simulink model "phi_mu"  (R2022a)
settings: Solver=VariableStepAuto  StartTime=0.0  StopTime=30  RelTol=1e-3
undefined symbols (not defined in the file or in its folder): G_phi_samples
libraries: simulink x4, cstblocks x2
settings Model: Creator=persian  LastModifiedBy=persian

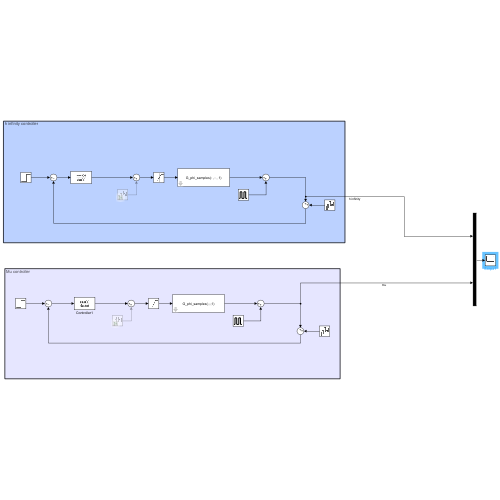
[thumbnail: Simulink's stored preview of the top-level diagram]
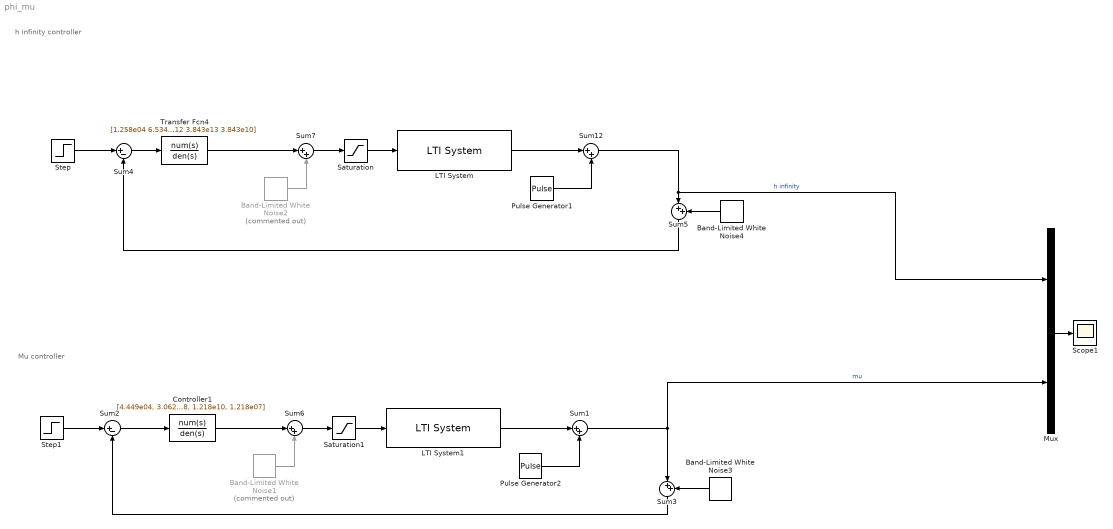
== system phi_mu ==
  note: h infinity controller
  note: Mu controller
  Band-Limited White Noise1 : simulink/Sources/Band-Limited White Noise  Commented=on  Cov=[0.001]  Ts=0.01  seed=[23341]
  Band-Limited White Noise2 : simulink/Sources/Band-Limited White Noise  Commented=on  Cov=[0.001]  Ts=0.01  seed=[23341]
  Band-Limited White Noise3 : simulink/Sources/Band-Limited White Noise  Cov=[0.0001]  Ts=0.01  seed=[23341]
  Band-Limited White Noise4 : simulink/Sources/Band-Limited White Noise  Cov=[0.0001]  Ts=0.01  seed=[23341]
  Controller1 : TransferFcn  Numerator=[4.449e04, 3.062e07, 8.69e08, 2.019e10, 1.453e11]  Denominator=[1, 3716, 2.98e06, 2.73e08, 1.218e10, 1.218e07]
  LTI System : cstblocks/LTI System  sys=G_phi_samples(: , : , 1)  IC=[]
  LTI System1 : cstblocks/LTI System  sys=G_phi_samples(:,:,1)  IC=[]
  Mux : Mux  Inputs=2
  Pulse Generator1 : DiscretePulseGenerator  PulseType=Time based  Amplitude=0.1  Period=1.5  PulseWidth=5
  Pulse Generator2 : DiscretePulseGenerator  PulseType=Time based  Amplitude=0.1  Period=1.5  PulseWidth=5
  Saturation : Saturate  UpperLimit=20  LowerLimit=-20
  Saturation1 : Saturate  UpperLimit=20  LowerLimit=-20
  Scope1 : Scope
  Step : Step  SampleTime=0
  Step1 : Step  SampleTime=0
  Sum{1,3,5..7,12} (6 alike) : Sum  Inputs=|++
  Sum2 : Sum  Inputs=|+-
  Sum4 : Sum  Inputs=|+-
  Transfer Fcn4 : TransferFcn  Numerator=[1.258e04 6.534e06 6.665e08 3.016e10 7.851e11 1.256e13 1.142e14 3.868e14]  Denominator=[1 2032 1.172e06 1.496e08 9.86e09 3.484e11 5.991e12 3.843e13 3.843e10]
  wires:
  Band-Limited White Noise1/1 -> Sum6/2
  Transfer Fcn4/1 -> Sum7/1
  Controller1/1 -> Sum6/1
  Band-Limited White Noise4/1 -> Sum5/2
  LTI System/1 -> Sum12/1
  Sum1/1 -> Mux/2, Sum3/1  "mu"
  Step/1 -> Sum4/1
  Band-Limited White Noise2/1 -> Sum7/2
  Sum7/1 -> Saturation/1
  Sum5/1 -> Sum4/2
  Sum4/1 -> Transfer Fcn4/1
  Sum12/1 -> Mux/1, Sum5/1  "h infinity"
  Sum3/1 -> Sum2/2
  Step1/1 -> Sum2/1
  Mux/1 -> Scope1/1
  Sum2/1 -> Controller1/1
  LTI System1/1 -> Sum1/1
  Saturation/1 -> LTI System/1
  Saturation1/1 -> LTI System1/1
  Band-Limited White Noise3/1 -> Sum3/2
  Pulse Generator1/1 -> Sum12/2
  Sum6/1 -> Saturation1/1
  Pulse Generator2/1 -> Sum1/2
